simulink library "LibEMIUtilities"  (Simulink 8.3)
settings: Solver=ode45  StartTime=0.0  StopTime=10.0  RelTol=1e-3
settings Model: Creator=swami  LastModifiedBy=swami

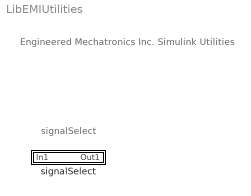
== system LibEMIUtilities ==
  note: signalSelect
  note: Engineered Mechatronics Inc. Simulink Utilities
  signalSelect : Subsystem  mask{signalSelectIndex=3}
      mask prompts: signalSelectIndex "Index (start at 1)"

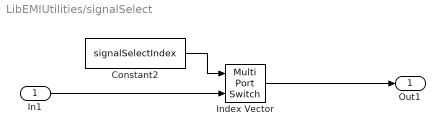
== system LibEMIUtilities/signalSelect ==
  In1 : Inport
  Constant2 : Constant  Value=signalSelectIndex
  Index Vector : MultiPortSwitch  Inputs=1
  Out1 : Outport
  wires:
  Constant2/1 -> Index Vector/1
  Index Vector/1 -> Out1/1
  In1/1 -> Index Vector/2
